simulink model "Ejemplo_filminas_simu"  (R2021a)
settings: Solver=VariableStepAuto  StartTime=0.0  StopTime=10.0  RelTol=1e-3
values from neighbouring files (symbols this model uses):
  A = [-2 -1; 0 -4]    [Control_Integral.m]    (also in Controlabilidad.m = P.a; Ejemplo_filminas.m = SS.A; Ejercicio_Inestable.m = [100, 0; 160, 200]; Ejercicio_Valvulas.m = double(A))
  B = [1; 0]    [Control_Integral.m]    (also in Controlabilidad.m = P.b; Ejemplo_filminas.m = SS.B; Ejercicio_Inestable.m = [70; 160]; Ejercicio_Valvulas.m = double(B))
  C = [1 1]    [Control_Integral.m]    (also in Controlabilidad.m = P.c; Ejemplo_filminas.m = SS.C; Ejercicio_Inestable.m = [1, 1]; Ejercicio_Valvulas.m = double(C))
  D = 0    [Control_Integral.m]    (also in Controlabilidad.m = P.d; Ejemplo_filminas.m = SS.D; Ejercicio_Inestable.m = 1; Ejercicio_Valvulas.m = double(D))
  K = [p1-a1 p2-a2] * Wrm * inv(Wr)    [Controlabilidad.m]    (also in Ejemplo_filminas.m; Ejercicio_Inestable.m = [p1 - a1, p2 - a2] * Wrm * inv(Wr); Ejercicio_Valvulas.m = Ka(1:order(P)); realimentacion_ee.m = acker(A, B, [-10 -10]))
  K_nuevo = Ka(1:order(P))    [Ejemplo_filminas.m]    (also in Ejercicio_Inestable.m = Ka(1:2))
  kf = -1/(C*inv(A - B*K) * B)    [Controlabilidad.m]    (also in Ejemplo_filminas.m = -1/(Ccl * inv(Acl)*Bcl); Ejercicio_Inestable.m = 1/(-(C - D*K) * inv(A - B*K) * B + D); realimentacion_ee.m = 10)
  ki = 10    [Control_Integral.m]    (also in Ejemplo_filminas.m = - Ka(end); Ejercicio_Inestable.m = - Ka(end); Ejercicio_Valvulas.m = - Ka(end))
settings Model: Creator=Santiago  LastModifiedBy=Santiago

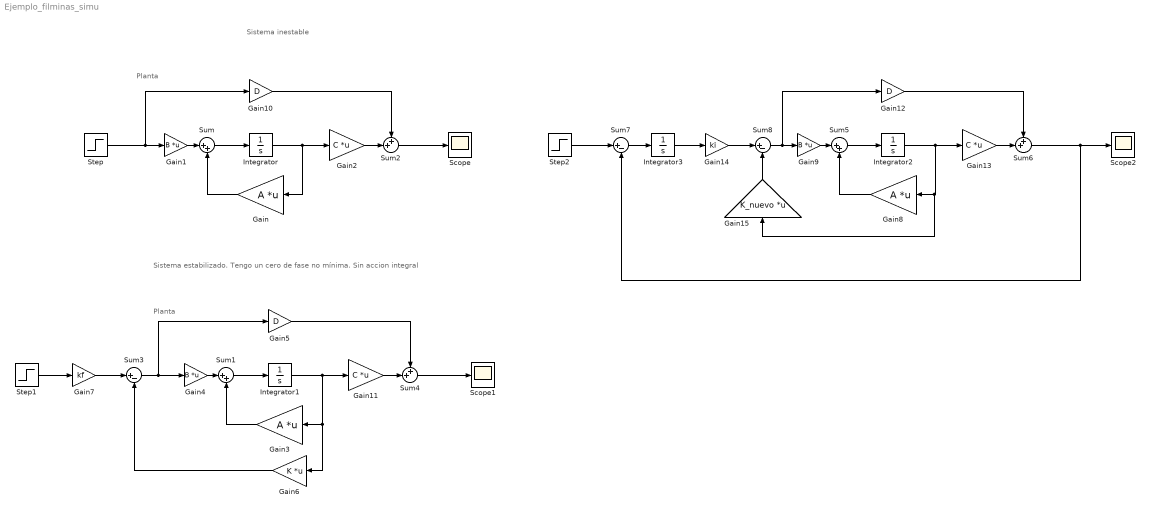
== system Ejemplo_filminas_simu ==
  note: Planta
  note: Sistema estabilizado. Tengo un cero de fase no mínima. Sin accion integral
  note: Planta
  note: Sistema inestable
  Gain : Gain  Gain=A  Multiplication=Matrix(K*u) (u vector)
  Gain1 : Gain  Gain=B  Multiplication=Matrix(K*u)
  Gain10 : Gain  Gain=D
  Gain11 : Gain  Gain=C  Multiplication=Matrix(K*u) (u vector)
  Gain12 : Gain  Gain=D
  Gain13 : Gain  Gain=C  Multiplication=Matrix(K*u) (u vector)
  Gain14 : Gain  Gain=ki
  Gain15 : Gain  Gain=K_nuevo  Multiplication=Matrix(K*u) (u vector)
  Gain2 : Gain  Gain=C  Multiplication=Matrix(K*u) (u vector)
  Gain3 : Gain  Gain=A  Multiplication=Matrix(K*u) (u vector)
  Gain4 : Gain  Gain=B  Multiplication=Matrix(K*u)
  Gain5 : Gain  Gain=D
  Gain6 : Gain  Gain=K  Multiplication=Matrix(K*u) (u vector)
  Gain7 : Gain  Gain=kf
  Gain8 : Gain  Gain=A  Multiplication=Matrix(K*u) (u vector)
  Gain9 : Gain  Gain=B  Multiplication=Matrix(K*u)
  Integrator{,1..3} (4 alike) : Integrator
  Scope : Scope
  Scope1 : Scope
  Scope2 : Scope
  Step : Step  SampleTime=0
  Step1 : Step  SampleTime=0
  Step2 : Step  SampleTime=0
  Sum : Sum  Inputs=|++
  Sum1 : Sum  Inputs=|++
  Sum2 : Sum  Inputs=++|
  Sum3 : Sum  Inputs=|+-
  Sum4 : Sum  Inputs=++|
  Sum5 : Sum  Inputs=|++
  Sum6 : Sum  Inputs=++|
  Sum7 : Sum  Inputs=|+-
  Sum8 : Sum  Inputs=|+-
  wires:
  Sum/1 -> Integrator/1
  Integrator/1 -> Gain/1, Gain2/1
  Gain/1 -> Sum/2
  Gain1/1 -> Sum/1
  Step/1 -> Gain10/1, Gain1/1
  Gain6/1 -> Sum3/2
  Step1/1 -> Gain7/1
  Gain7/1 -> Sum3/1
  Gain10/1 -> Sum2/1
  Gain2/1 -> Sum2/2
  Sum2/1 -> Scope/1
  Sum4/1 -> Scope1/1
  Gain11/1 -> Sum4/2
  Gain5/1 -> Sum4/1
  Sum1/1 -> Integrator1/1
  Gain3/1 -> Sum1/2
  Gain4/1 -> Sum1/1
  Integrator1/1 -> Gain6/1, Gain3/1, Gain11/1
  Sum3/1 -> Gain5/1, Gain4/1
  Sum6/1 -> Sum7/2, Scope2/1
  Gain13/1 -> Sum6/2
  Gain12/1 -> Sum6/1
  Gain8/1 -> Sum5/2
  Sum5/1 -> Integrator2/1
  Gain9/1 -> Sum5/1
  Integrator2/1 -> Gain15/1, Gain8/1, Gain13/1
  Gain15/1 -> Sum8/2
  Step2/1 -> Sum7/1
  Sum7/1 -> Integrator3/1
  Integrator3/1 -> Gain14/1
  Gain14/1 -> Sum8/1
  Sum8/1 -> Gain12/1, Gain9/1
